simulink model "MSAP"  (R2019b)
settings: Solver=VariableStepAuto  StartTime=0.0  StopTime=2  RelTol=1e-3  EnableMultiTasking=on
values from neighbouring files (symbols this model uses):
  A = [0 -Lq; Ld 0]    [Para_MSAP.m]
  F = 0.59e-4    (= 5.9e-05)    [Para_MSAP.m]
  J = 0.9    [Para_MSAP.m]
  L = [Ld 0; 0 Lq]    [Para_MSAP.m]
  P = 2    [Para_MSAP.m]
  PhiF = [0 ; Phi_n]    [Para_MSAP.m]
  R = [Rs 0; 0 Rs]    [Para_MSAP.m]
settings Model: Creator=User  LastModifiedBy=x1 yoga
settings DataIOCC: ReturnWorkspaceOutputs=off
settings OptimizationCC: LifeSpan=inf
settings DebuggingCC: SFUnexpectedBacktrackingDiag=warning  SFNoUnconditionalDefaultTransitionDiag=warning  ArithmeticOperatorsInVariantConditions=warning
settings SFSimCC: SimUseLocalCustomCode=off  CustomCodeUndefinedFunction=UseInterfaceOnly
settings RTWCC: RTWUseLocalCustomCode=off
settings CodeAppCC: StateflowObjectComments=on
settings GRTTargetCC: TargetLangStandard=C89/C90 (ANSI)  GeneratePreprocessorConditionals=Disable all
settings ConfigComp: CovMetricSettings=dw  CovHtmlReporting=on  CovSaveCumulativeToWorkspaceVar=on  CovSaveSingleToWorkspaceVar=on  CovExternalEMLEnable=off

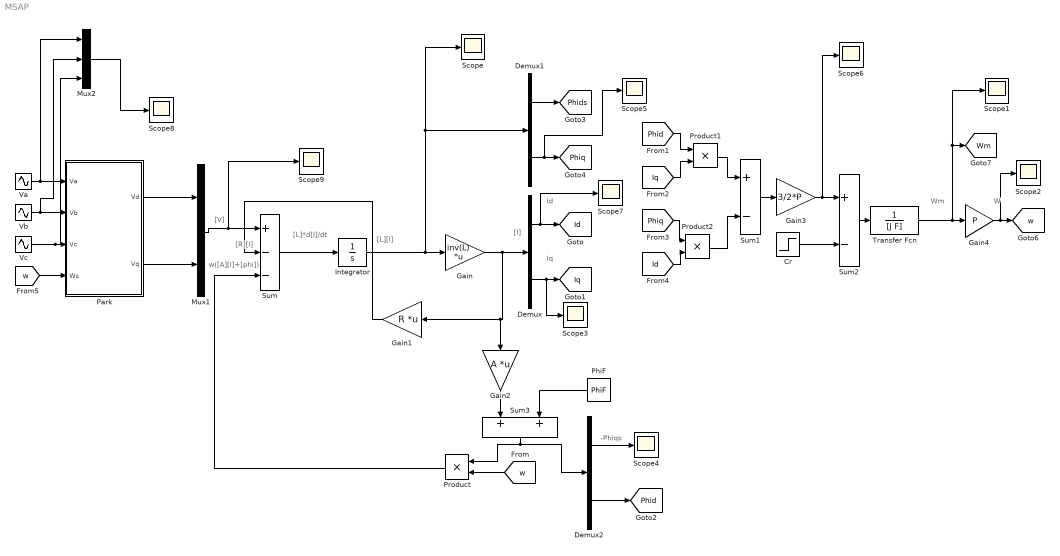
== system MSAP ==
  note: -Phiqs
  note: W
  note: Wm
  note: Iq
  note: Id
  note: [I]
  note: [L][I]
  note: [L]*d[I]/dt
  note: w([A][I]+[phi])
  note: [R][I]
  note: [V]
  Cr : Step  Time=2  Before=0.4  After=5  SampleTime=0
  Demux : Demux  Outputs=2
  Demux1 : Demux  Outputs=2
  Demux2 : Demux  Outputs=2
  Gain : Gain  Gain=inv(L)  Multiplication=Matrix(K*u)  LockScale=on
  Gain1 : Gain  Gain=R  Multiplication=Matrix(K*u)  LockScale=on
  Gain2 : Gain  Gain=A  Multiplication=Matrix(K*u)  LockScale=on
  Gain3 : Gain  Gain=3/2*P  LockScale=on
  Gain4 : Gain  Gain=P  LockScale=on
  Integrator : Integrator
  Mux1 : Mux  Inputs=2
  Mux2 : Mux  Inputs=3
  Park : Subsystem
  PhiF : Constant  Value=PhiF  LockScale=on
  Product : Product
  Product1 : Product
  Product2 : Product
  Scope{,1..9} (10 alike) : Scope
  Sum : Sum  Inputs=+--
  Sum1 : Sum  Inputs=+-
  Sum2 : Sum  Inputs=+-
  Sum3 : Sum
  Transfer Fcn : TransferFcn  Denominator=[J F]
  Va : Sin  Amplitude=141  Frequency=2*pi*50  SampleTime=0
  Vb : Sin  Amplitude=141  Frequency=2*pi*50  Phase=-2*pi/3  SampleTime=0
  Vc : Sin  Amplitude=141  Frequency=2*pi*50  Phase=2*pi/3  SampleTime=0
  tag scope: Id=global, Iq=global, Phid=global, Phids=global, Phiq=global, Wm=global, w=global
  wires:
  Va/1 -> Mux2/1, Park/1(Va)
  Vb/1 -> Mux2/2, Park/2(Vb)
  Vc/1 -> Mux2/3, Park/3(Vc)
  [w] -> Park/4(Ws)
  Park/1("Vd ") -> Mux1/1
  Park/2("Vq ") -> Mux1/2
  Mux1/1 -> Scope9/1, Sum/1
  Sum/1 -> Integrator/1
  Integrator/1 -> Scope/1, Demux1/1, Gain/1
  Gain/1 -> Gain1/1, Gain2/1, Demux/1
  Gain1/1 -> Sum/2
  [w] -> Product/2
  Demux/1 -> [Id], Scope7/1
  Demux/2 -> Scope3/1, [Iq]
  Demux1/2 -> Scope5/1, [Phiq]
  [Phid] -> Product1/1
  [Iq] -> Product1/2
  [Phiq] -> Product2/1
  [Id] -> Product2/2
  Product1/1 -> Sum1/1
  Product2/1 -> Sum1/2
  Sum1/1 -> Gain3/1
  Gain3/1 -> Scope6/1, Sum2/1
  Sum2/1 -> Transfer Fcn/1
  Cr/1 -> Sum2/2
  Transfer Fcn/1 -> Gain4/1, Scope1/1, [Wm]
  Gain4/1 -> Scope2/1, [w]
  Demux1/1 -> [Phids]
  Gain2/1 -> Sum3/1
  Sum3/1 -> Demux2/1, Product/1
  Product/1 -> Sum/3
  PhiF/1 -> Sum3/2
  Demux2/2 -> [Phid]
  Demux2/1 -> Scope4/1
  Mux2/1 -> Scope8/1

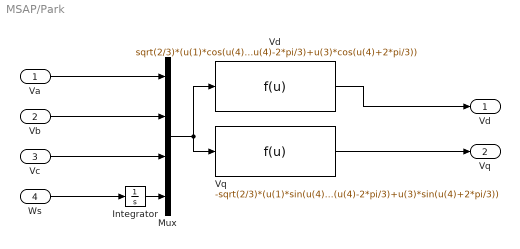
== system MSAP/Park ==
  Va : Inport
  Vb : Inport  Port=2
  Vc : Inport  Port=3
  Ws : Inport  Port=4
  Integrator : Integrator
  Mux : Mux
  Vd : Fcn  Expr=sqrt(2/3)*(u(1)*cos(u(4))+u(2)*cos(u(4)-2*pi/3)+u(3)*cos(u(4)+2*pi/3))
  Vq : Fcn  Expr=-sqrt(2/3)*(u(1)*sin(u(4))+u(2)*sin(u(4)-2*pi/3)+u(3)*sin(u(4)+2*pi/3))
  "Vd " : Outport
  "Vq " : Outport  Port=2
  wires:
  Vq/1 -> "Vq "/1
  Vd/1 -> "Vd "/1
  Vb/1 -> Mux/2
  Ws/1 -> Integrator/1
  Integrator/1 -> Mux/4
  Mux/1 -> Vq/1, Vd/1
  Va/1 -> Mux/1
  Vc/1 -> Mux/3
